simulink model "test_of_traj"  (R2015a)
settings: Solver=ode45  StartTime=0.0  StopTime=40  RelTol=1e-3
undefined symbols (not defined in the file or in its folder): fuzzy_DM
libraries: simulink x3, fuzblock x1
settings Model: Creator=Oussama  LastModifiedBy=Oussama

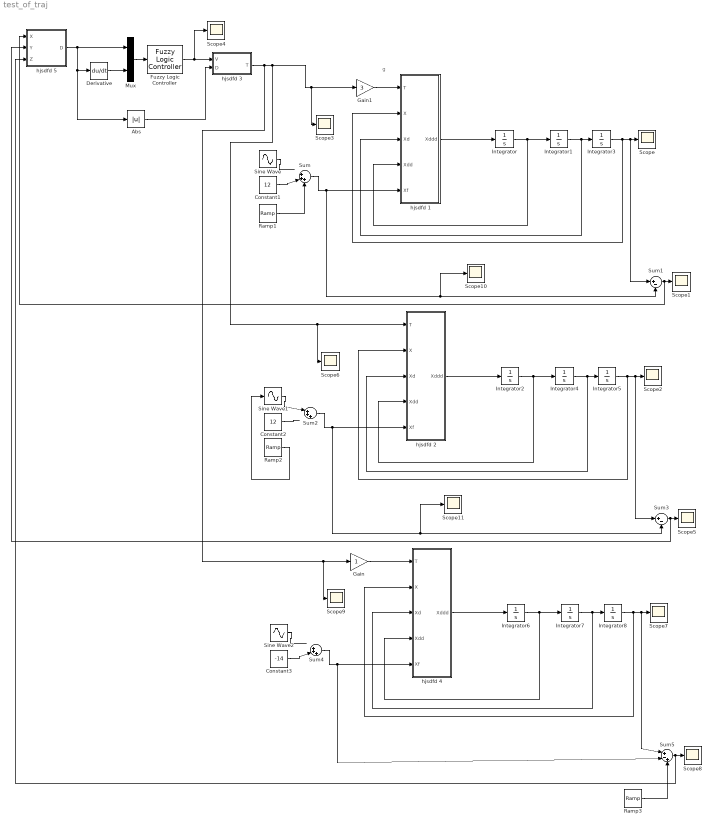
== system test_of_traj ==
  note: g
  Abs : Abs
  Constant1 : Constant  Value=12
  Constant2 : Constant  Value=12
  Constant3 : Constant  Value=-14
  Derivative : Derivative
  Fuzzy Logic Controller : fuzblock/Fuzzy Logic  Controller  fis=[fuzzy_DM]
  Gain : Gain
  Gain1 : Gain  Gain=3
  Integrator{,1..8} (9 alike) : Integrator
  Mux : Mux  Inputs=2
  Ramp1 : simulink/Sources/Ramp  slope=0.35  start=0  X0=0
  Ramp2 : simulink/Sources/Ramp  slope=1  start=0  X0=0
  Ramp3 : simulink/Sources/Ramp  slope=50  start=15  X0=0
  Scope{,1..11} (12 alike) : Scope
      Scope settings: TimeRange=6.132805158380197  YMin=11.783203125  YMax=12.228515625  SaveName=X
      Scope1 settings: TimeRange=6.132805158380197  YMin=11.783203125  YMax=12.228515625
      Scope10 settings: TimeRange=6.132805158380197  YMin=11.783203125  YMax=12.228515625  SaveName=XX
      Scope11 settings: TimeRange=6.132805158380197  YMin=11.783203125  YMax=12.228515625  SaveName=YY
      Scope2 settings: TimeRange=6.132805158380197  YMin=11.783203125  YMax=12.228515625  SaveName=Y
      Scope3 settings: TimeRange=6.132805158380197  YMin=11.783203125  YMax=12.228515625  SaveName=ScopeData3
      Scope4 settings: TimeRange=6.132805158380197  YMin=11.783203125  YMax=12.228515625  SaveName=ScopeData4
      Scope5 settings: TimeRange=6.132805158380197  YMin=11.783203125  YMax=12.228515625  SaveName=ScopeData5
      Scope6 settings: TimeRange=6.132805158380197  YMin=11.783203125  YMax=12.228515625  SaveName=ScopeData6
      Scope7 settings: TimeRange=6.132805158380197  YMin=11.783203125  YMax=12.228515625  SaveName=Z
      Scope8 settings: TimeRange=6.132805158380197  YMin=11.783203125  YMax=12.228515625  SaveName=ScopeData8
      Scope9 settings: TimeRange=6.132805158380197  YMin=11.783203125  YMax=12.228515625  SaveName=ScopeData9
  Sine Wave : Sin  SampleTime=0
  Sine Wave1 : Sin  TimeSource=Use external signal  Frequency=0.35  SampleTime=0
  Sine Wave2 : Sin  SampleTime=0
  Sum : Sum  Inputs=|+++
  Sum1 : Sum  Inputs=|+-
  Sum2 : Sum  Inputs=|+++
  Sum3 : Sum  Inputs=|+-
  Sum4 : Sum  Inputs=|+++
  Sum5 : Sum  Inputs=|+-+
  hjsdfd 1 : MATLAB Function  TreatAsAtomicUnit=on
  hjsdfd 2 : MATLAB Function  TreatAsAtomicUnit=on
  hjsdfd 3 : MATLAB Function  TreatAsAtomicUnit=on
  hjsdfd 4 : MATLAB Function  TreatAsAtomicUnit=on
  hjsdfd 5 : MATLAB Function  TreatAsAtomicUnit=on
  wires:
  Integrator/1 -> hjsdfd 1/4(Xdd), Integrator1/1
  Integrator1/1 -> hjsdfd 1/3(Xd), Integrator3/1
  Integrator3/1 -> hjsdfd 1/2(X), Sum1/1, Scope/1
  hjsdfd 1/1(Xddd) -> Integrator/1
  Constant1/1 -> Sum/2
  Sum/1 -> Scope10/1, Sum1/2, hjsdfd 1/5(Xf)
  Sum1/1 -> hjsdfd 5/1(X), Scope1/1
  Ramp1/1 -> Sum/3
  Sine Wave/1 -> ?
  Mux/1 -> Fuzzy Logic Controller/1
  Derivative/1 -> Mux/2
  Fuzzy Logic Controller/1 -> Scope4/1, hjsdfd 3/1(V)
  Abs/1 -> hjsdfd 3/2(D)
  Integrator2/1 -> hjsdfd 2/4(Xdd), Integrator4/1
  Integrator4/1 -> hjsdfd 2/3(Xd), Integrator5/1
  Integrator5/1 -> hjsdfd 2/2(X), Sum3/1, Scope2/1
  hjsdfd 2/1(Xddd) -> Integrator2/1
  Constant2/1 -> ?
  Sum2/1 -> Scope11/1, Sum3/2, hjsdfd 2/5(Xf)
  Ramp2/1 -> Sine Wave1/1
  Sine Wave1/1 -> Sum2/1
  hjsdfd 3/1(T) -> Gain/1, Scope9/1, hjsdfd 2/1(T), Scope6/1, Gain1/1, Scope3/1
  Integrator6/1 -> hjsdfd 4/4(Xdd), Integrator7/1
  Integrator7/1 -> hjsdfd 4/3(Xd), Integrator8/1
  Integrator8/1 -> hjsdfd 4/2(X), Sum5/1, Scope7/1
  hjsdfd 4/1(Xddd) -> Integrator6/1
  Constant3/1 -> Sum4/2
  Sum4/1 -> Sum5/2, hjsdfd 4/5(Xf)
  Ramp3/1 -> Sum5/3
  Sine Wave2/1 -> ?
  hjsdfd 5/1(D) -> Abs/1, Derivative/1, Mux/1
  Sum3/1 -> hjsdfd 5/2(Y), Scope5/1
  Sum5/1 -> hjsdfd 5/3(Z), Scope8/1
  Gain/1 -> hjsdfd 4/1(T)
  Gain1/1 -> hjsdfd 1/1(T)

== matlab function test_of_traj/hjsdfd 2 ==
  data: T input; Xddd output; X input; Xd input; Xdd input; Xf input
function Xddd  = fcn(T,X, Xd,Xdd,Xf )

Xddd= -60/T^3*X - 36/T^2 * Xd -9 /T * Xdd + 60 /T^3 * Xf;

== matlab function test_of_traj/hjsdfd 3 ==
  data: T output; V input; D input
function T  = fcn(V,D)

T= D/V+0.5;

== matlab function test_of_traj/hjsdfd 4 ==
  data: T input; Xddd output; X input; Xd input; Xdd input; Xf input
function Xddd  = fcn(T,X, Xd,Xdd,Xf )

Xddd= -60/T^3*X - 36/T^2 * Xd -9 /T * Xdd + 60 /T^3 * Xf;

== matlab function test_of_traj/hjsdfd 5 ==
  data: X input; D output; Y input; Z input
function D  = fcn(X,Y,Z)

D= sqrt(X^2+Y^2);

== matlab function test_of_traj/hjsdfd 1 ==
  data: T input; Xddd output; X input; Xd input; Xdd input; Xf input
function Xddd  = fcn(T,X, Xd,Xdd,Xf )

Xddd= -60/T^3*X - 36/T^2 * Xd -9 /T * Xdd + 60 /T^3 * Xf;
